simulink model "Lcontainer_simNN"  (R2018b)
settings: Solver=FixedStepAuto  StartTime=0.0  StopTime=600  FixedStep=0.1  RelTol=1e-3
libraries: neural x88, simulink x1
(part 3 of 4)

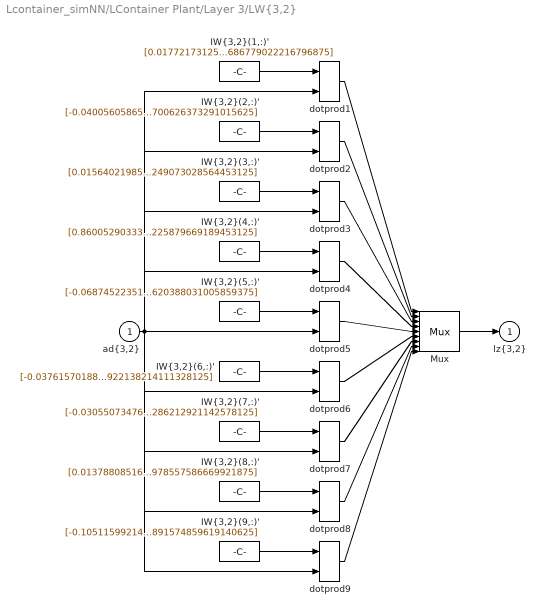
== system Lcontainer_simNN/LContainer Plant/Layer 3/LW{3,2} ==
  "ad{3,2}" : Inport  PortDimensions=10
      mask Display: e = 0.06;c1 = [120 230 180]/255;c2 = ([120 230 180]+0)/(256+128);c3 = ([120 230 180]+128)/(256+128);patch([0 1 1 0],[0 0 1 1],c1);patch([0 1 1 1-e 1-e 0+e],[0 0 1 1-e 0+e 0+e],c2);patch([0 0 1 1-e 0+e 0+e],[0 1 1 1-e 1-e 0+e],c3);plot([0 1 1 0 0],[0 0 1 1 0]);
  "IW{3,2}(1,:)'" : Constant  Value=[0.017721731250787138567392986487902817316353321075439453125;3.000123587276951301099561015566332824954398723004377058654057464082143269479274749755859375e-18;0.006631368793965075440766110403956190566532313823699951171875;0.0005830819266561507348278770024307959829457104206085205078125;-0.00058009248650328962791655751374264582409523427486419677734375;0.00089743107072331150531052657015607110224664211273193359375;0.000417621773328847646113148872615283835330046713352203369140625;-2.208352547409586067716440764973830234430475893202518079155068780883297563377709593623876571655273438e-21;0.00013978297890123654351364479442310084778000600636005401611328125;0.000674010021193850554499515936868192511610686779022216796875]
      mask Display: e = 0.06;c1 = [120 150 230]/255;c2 = ([120 150 230]+0)/383;c3 = ([120 150 230]+128)/383;patch([0 1 1 0],[0 0 1 1],c1);patch([0 1 1 1-e 1-e 0+e],[0 0 1 1-e 0+e 0+e],c2);patch([0 0 1 1-e 0+e 0+e],[0 1 1 1-e 1-e 0+e],c3);plot([0 1 1 0 0],[0 0 1 1 0]);disp('weights');
  "IW{3,2}(2,:)'" : Constant  Value=[-0.04005605865106844076795056253104121424257755279541015625;-3.29867064884893000845695736657715495575445867532972388236345295808860100805759429931640625e-17;0.06916512907204268312266748353067669086158275604248046875;-0.042226033791083257551424168241283041425049304962158203125;0.034903285783379846274332436451004468835890293121337890625;-0.0021373573678505207625033524010405017179436981678009033203125;-0.003622572133452827032595866540987117332406342029571533203125;2.9787149770187764768538925291780095327185039558298075188479125952056847381754778325557708740234375e-22;0.0435714010459078426862333799363113939762115478515625;0.000252495443577469718711425716861640466959215700626373291015625]
      mask Display: e = 0.06;c1 = [120 150 230]/255;c2 = ([120 150 230]+0)/383;c3 = ([120 150 230]+128)/383;patch([0 1 1 0],[0 0 1 1],c1);patch([0 1 1 1-e 1-e 0+e],[0 0 1 1-e 0+e 0+e],c2);patch([0 0 1 1-e 0+e 0+e],[0 1 1 1-e 1-e 0+e],c3);plot([0 1 1 0 0],[0 0 1 1 0]);disp('weights');
  "IW{3,2}(3,:)'" : Constant  Value=[0.0156402198576308069932760957954087643884122371673583984375;-2.7705357247132681851359167346903580323963177435846357010706952905820799060165882110595703125e-17;0.005717664581344373588012164333349574008025228977203369140625;0.001120727306336578681100757393096500891260802745819091796875;-0.0010906626797669602239870823012779510463587939739227294921875;0.000717501659741846928471098454593857240979559719562530517578125;0.00049104555462250770898890994686780686606653034687042236328125;-8.808503989752254956010719320420912897565545125168497871668595033955995177166187204420566558837890625e-22;0.00025255883377770980101340025925082954927347600460052490234375;-0.00104828749438158792817166187205657479353249073028564453125]
      mask Display: e = 0.06;c1 = [120 150 230]/255;c2 = ([120 150 230]+0)/383;c3 = ([120 150 230]+128)/383;patch([0 1 1 0],[0 0 1 1],c1);patch([0 1 1 1-e 1-e 0+e],[0 0 1 1-e 0+e 0+e],c2);patch([0 0 1 1-e 0+e 0+e],[0 1 1 1-e 1-e 0+e],c3);plot([0 1 1 0 0],[0 0 1 1 0]);disp('weights');
  "IW{3,2}(4,:)'" : Constant  Value=[0.86005290333067818675516491566668264567852020263671875;1.08054859226237535721582342014765368435526095617325859077340055591776035726070404052734375e-16;0.4392103630130466118686172194429673254489898681640625;0.0309526769540591877027946310363404336385428905487060546875;-0.030153085840038874876345431630397797562181949615478515625;0.025833991374961805254084623584276414476335048675537109375;-0.0286867731698114518390507754475038382224738597869873046875;1.04433448485527096216197080488959096762601167281087898865664376213402420034981332719326019287109375e-20;0.01039470392753527594464912908733822405338287353515625;-0.00160357287137106942383202312640833042678423225879669189453125]
      mask Display: e = 0.06;c1 = [120 150 230]/255;c2 = ([120 150 230]+0)/383;c3 = ([120 150 230]+128)/383;patch([0 1 1 0],[0 0 1 1],c1);patch([0 1 1 1-e 1-e 0+e],[0 0 1 1-e 0+e 0+e],c2);patch([0 0 1 1-e 0+e 0+e],[0 1 1 1-e 1-e 0+e],c3);plot([0 1 1 0 0],[0 0 1 1 0]);disp('weights');
  "IW{3,2}(5,:)'" : Constant  Value=[-0.0687452235173775239029936301449197344481945037841796875;-2.0902295329942603015523256376234939712702367786635766766512034564584610052406787872314453125e-17;-0.1778346260095364506081949684812570922076702117919921875;0.37951707531323919386778698026319034397602081298828125;-0.25677471515412253477705917248385958373546600341796875;0.282905692872918612668087234851554967463016510009765625;0.28903582809806682707431946255383081734180450439453125;1.168985956367130130783772982847233629991089391960804043152279824147043996163120027631521224975585938e-21;0.298430584822482192208781270892359316349029541015625;0.270396007685359263117419459376833401620388031005859375]
      mask Display: e = 0.06;c1 = [120 150 230]/255;c2 = ([120 150 230]+0)/383;c3 = ([120 150 230]+128)/383;patch([0 1 1 0],[0 0 1 1],c1);patch([0 1 1 1-e 1-e 0+e],[0 0 1 1-e 0+e 0+e],c2);patch([0 0 1 1-e 0+e 0+e],[0 1 1 1-e 1-e 0+e],c3);plot([0 1 1 0 0],[0 0 1 1 0]);disp('weights');
  "IW{3,2}(6,:)'" : Constant  Value=[-0.037615701889427345661065515969312400557100772857666015625;-2.0255214901096142112965294281557460666901378224425030183386553517266293056309223175048828125e-17;-0.018940509565756220855536895442128297872841358184814453125;-0.0011494809468569548542571379101673301192931830883026123046875;0.0003933836267355390338938680994118612943566404283046722412109375;-0.00270488027420923322907686525695680757053196430206298828125;-0.0035495085585161519937946739133849405334331095218658447265625;2.771026078124981596591574202811655532744747077067631470356952327893651499834959395229816436767578125e-21;-0.005884709230925987653859632331432294449768960475921630859375;-0.002282368848335381006364741551806218922138214111328125]
      mask Display: e = 0.06;c1 = [120 150 230]/255;c2 = ([120 150 230]+0)/383;c3 = ([120 150 230]+128)/383;patch([0 1 1 0],[0 0 1 1],c1);patch([0 1 1 1-e 1-e 0+e],[0 0 1 1-e 0+e 0+e],c2);patch([0 0 1 1-e 0+e 0+e],[0 1 1 1-e 1-e 0+e],c3);plot([0 1 1 0 0],[0 0 1 1 0]);disp('weights');
  "IW{3,2}(7,:)'" : Constant  Value=[-0.0305507347678967249027248698212133604101836681365966796875;2.7496360392653631819364899496901638274924214552417077450652271863873465918004512786865234375e-17;0.0037154083625400755562517840502323451801203191280364990234375;-0.0117954745462954015133849594576531671918928623199462890625;0.00873441603258174291413151735241626738570630550384521484375;-0.00256346476134278015990286547776122461073100566864013671875;-0.0002901674951942543917611516679500027748872525990009307861328125;2.874094316443142059162815388265592867958623516934298226354737443299924848361115437000989913940429688e-21;0.009189198861728177514240911705201142467558383941650390625;-0.0149119845092046850176803474141706828959286212921142578125]
      mask Display: e = 0.06;c1 = [120 150 230]/255;c2 = ([120 150 230]+0)/383;c3 = ([120 150 230]+128)/383;patch([0 1 1 0],[0 0 1 1],c1);patch([0 1 1 1-e 1-e 0+e],[0 0 1 1-e 0+e 0+e],c2);patch([0 0 1 1-e 0+e 0+e],[0 1 1 1-e 1-e 0+e],c3);plot([0 1 1 0 0],[0 0 1 1 0]);disp('weights');
  "IW{3,2}(8,:)'" : Constant  Value=[0.01378808516196154514144023295330043765716254711151123046875;-4.899238598294270608298336688091797164883411976597261949795125701712095178663730621337890625e-17;-0.02461851504914606969531831737185711972415447235107421875;0.053656095043096409258343015835635014809668064117431640625;-0.06243497389268269637252473103217198513448238372802734375;-0.006117530417972946547855439547447531367652118206024169921875;0.005742975335650324364422658618423156440258026123046875;-1.090939145799021708153406170841651324421968177498445589848749190386989482703938847407698631286621094e-21;-0.00137001382693252723131427384117841938859783113002777099609375;0.03560214339080740308940420391081715933978557586669921875]
      mask Display: e = 0.06;c1 = [120 150 230]/255;c2 = ([120 150 230]+0)/383;c3 = ([120 150 230]+128)/383;patch([0 1 1 0],[0 0 1 1],c1);patch([0 1 1 1-e 1-e 0+e],[0 0 1 1-e 0+e 0+e],c2);patch([0 0 1 1-e 0+e 0+e],[0 1 1 1-e 1-e 0+e],c3);plot([0 1 1 0 0],[0 0 1 1 0]);disp('weights');
  "IW{3,2}(9,:)'" : Constant  Value=[-0.10511599214514828759536868574286927469074726104736328125;5.121980772139466446942862502458263931975946490625546669850365333331865258514881134033203125e-17;0.2601261896053455036081913931411691009998321533203125;-0.136425741683425361117087959428317844867706298828125;0.1081606731296494150473819217950222082436084747314453125;-0.0089247157820076909728879144267921219579875469207763671875;0.0011455689908133749425889202910866515594534575939178466796875;8.549650359076011053606725543058816108935553021266017400495596662013397804003034252673387527465820313e-22;0.1629678156227741536721254078656784258782863616943359375;0.83692845002217597372151658419170416891574859619140625]
      mask Display: e = 0.06;c1 = [120 150 230]/255;c2 = ([120 150 230]+0)/383;c3 = ([120 150 230]+128)/383;patch([0 1 1 0],[0 0 1 1],c1);patch([0 1 1 1-e 1-e 0+e],[0 0 1 1-e 0+e 0+e],c2);patch([0 0 1 1-e 0+e 0+e],[0 1 1 1-e 1-e 0+e],c3);plot([0 1 1 0 0],[0 0 1 1 0]);disp('weights');
  Mux : Mux  Inputs=9
      mask Display: e = 0.06;c1 = [120 150 230]/255;c2 = ([120 150 230]+0)/383;c3 = ([120 150 230]+128)/383;patch([0 1 1 0],[0 0 1 1],c1);patch([0 1 1 1-e 1-e 0+e],[0 0 1 1-e 0+e 0+e],c2);patch([0 0 1 1-e 0+e 0+e],[0 1 1 1-e 1-e 0+e],c3);plot([0 1 1 0 0],[0 0 1 1 0]);disp('Mux');
  dotprod{1..9} (9 alike) : neural/Weight Functions/dotprod
  "lz{3,2}" : Outport
      mask Display: e = 0.06;c1 = [120 230 180]/255;c2 = ([120 230 180]+0)/(256+128);c3 = ([120 230 180]+128)/(256+128);patch([0 1 1 0],[0 0 1 1],c1);patch([0 1 1 1-e 1-e 0+e],[0 0 1 1-e 0+e 0+e],c2);patch([0 0 1 1-e 0+e 0+e],[0 1 1 1-e 1-e 0+e],c3);plot([0 1 1 0 0],[0 0 1 1 0]);
  wires:
  Mux/1 -> "lz{3,2}"/1
  dotprod9/1 -> Mux/9
  "IW{3,2}(9,:)'"/1 -> dotprod9/1
  dotprod8/1 -> Mux/8
  "IW{3,2}(8,:)'"/1 -> dotprod8/1
  dotprod7/1 -> Mux/7
  "IW{3,2}(7,:)'"/1 -> dotprod7/1
  dotprod6/1 -> Mux/6
  "IW{3,2}(6,:)'"/1 -> dotprod6/1
  dotprod5/1 -> Mux/5
  "IW{3,2}(5,:)'"/1 -> dotprod5/1
  dotprod4/1 -> Mux/4
  "IW{3,2}(4,:)'"/1 -> dotprod4/1
  dotprod3/1 -> Mux/3
  "IW{3,2}(3,:)'"/1 -> dotprod3/1
  dotprod2/1 -> Mux/2
  "IW{3,2}(2,:)'"/1 -> dotprod2/1
  dotprod1/1 -> Mux/1
  "ad{3,2}"/1 -> dotprod9/2, dotprod8/2, dotprod7/2, dotprod6/2, dotprod5/2, dotprod4/2, dotprod3/2, dotprod2/2, dotprod1/2
  "IW{3,2}(1,:)'"/1 -> dotprod1/1

== system Lcontainer_simNN/LContainer tr/Layer 1/Delays 1 ==
  "p{1}" : Inport  PortDimensions=19
      mask Display: e = 0.06;c1 = [120 230 180]/255;c2 = ([120 230 180]+0)/(256+128);c3 = ([120 230 180]+128)/(256+128);patch([0 1 1 0],[0 0 1 1],c1);patch([0 1 1 1-e 1-e 0+e],[0 0 1 1-e 0+e 0+e],c2);patch([0 0 1 1-e 0+e 0+e],[0 1 1 1-e 1-e 0+e],c3);plot([0 1 1 0 0],[0 0 1 1 0]);
  mux : Mux  Inputs=1
      mask Display: e = 0.06;c1 = [120 150 230]/255;c2 = ([120 150 230]+0)/383;c3 = ([120 150 230]+128)/383;patch([0 1 1 0],[0 0 1 1],c1);patch([0 1 1 1-e 1-e 0+e],[0 0 1 1-e 0+e 0+e],c2);patch([0 0 1 1-e 0+e 0+e],[0 1 1 1-e 1-e 0+e],c3);plot([0 1 1 0 0],[0 0 1 1 0]);disp('Mux')
  "pd{1,1}" : Outport
      mask Display: e = 0.06;c1 = [120 230 180]/255;c2 = ([120 230 180]+0)/(256+128);c3 = ([120 230 180]+128)/(256+128);patch([0 1 1 0],[0 0 1 1],c1);patch([0 1 1 1-e 1-e 0+e],[0 0 1 1-e 0+e 0+e],c2);patch([0 0 1 1-e 0+e 0+e],[0 1 1 1-e 1-e 0+e],c3);plot([0 1 1 0 0],[0 0 1 1 0]);
  wires:
  mux/1 -> "pd{1,1}"/1
  "p{1}"/1 -> mux/1

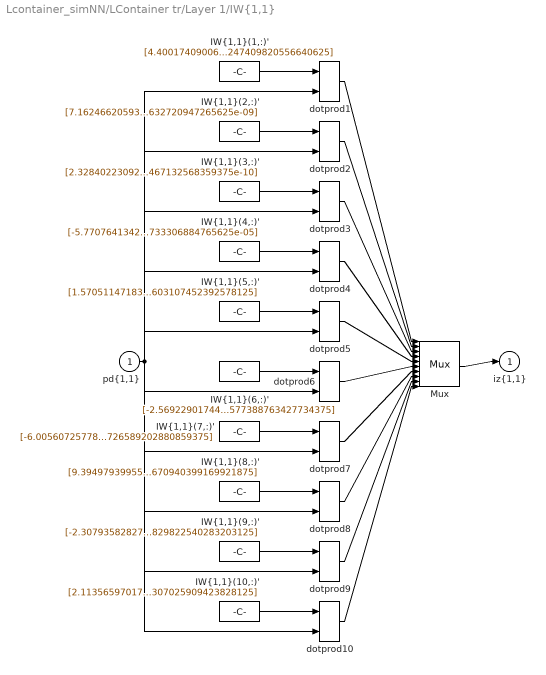
== system Lcontainer_simNN/LContainer tr/Layer 1/IW{1,1} ==
  "pd{1,1}" : Inport  PortDimensions=19
      mask Display: e = 0.06;c1 = [120 230 180]/255;c2 = ([120 230 180]+0)/(256+128);c3 = ([120 230 180]+128)/(256+128);patch([0 1 1 0],[0 0 1 1],c1);patch([0 1 1 1-e 1-e 0+e],[0 0 1 1-e 0+e 0+e],c2);patch([0 0 1 1-e 0+e 0+e],[0 1 1 1-e 1-e 0+e],c3);plot([0 1 1 0 0],[0 0 1 1 0]);
  "IW{1,1}(1,:)'" : Constant  Value=[4.40017409006617107452076869647701606869105717123602516949176788330078125e-09;0.01345267619395669640713908421503219869919121265411376953125;8.158769329916370116780044430271345845540054142475128173828125e-05;0.133282506165966319056082056704326532781124114990234375;0.118798799147599110082040851921192370355129241943359375;-0.00160146802195825096147563382231737705296836793422698974609375;0.00361362526321039496945974889285935205407440662384033203125;0.00402460725956179689311031921761241392232477664947509765625;0.1388328803151288315387290595026570372283458709716796875;0.13563305647747092574917360252584330737590789794921875;0.03992381222266881690696749274138710461556911468505859375;-0.0016005219135142756577139255824704378028400242328643798828125;0.433616038493515876250938845259952358901500701904296875;0.48731317755691783144555984108592383563518524169921875;0.0112602065374665973040979594088639714755117893218994140625;0.004024609800961928031404202243948020623065531253814697265625;-0.07276424533892690560410443367800326086580753326416015625;-0.036403357952666894059579050235697650350630283355712890625;0.0019376179722031734199705343968389570363797247409820556640625]
      mask Display: e = 0.06;c1 = [120 150 230]/255;c2 = ([120 150 230]+0)/383;c3 = ([120 150 230]+128)/383;patch([0 1 1 0],[0 0 1 1],c1);patch([0 1 1 1-e 1-e 0+e],[0 0 1 1-e 0+e 0+e],c2);patch([0 0 1 1-e 0+e 0+e],[0 1 1 1-e 1-e 0+e],c3);plot([0 1 1 0 0],[0 0 1 1 0]);disp('Weights');
  "IW{1,1}(10,:)'" : Constant  Value=[2.113565970177129623007061133470947840440334886125128832645714282989501953125e-10;0.03896513174368167187200384660172858275473117828369140625;-0.00069289406221726963612528304992110861348919570446014404296875;-0.00762248639883274237138977014183183200657367706298828125;0.383227265395797156433133068276220001280307769775390625;-0.0034013008372572842326342357210933187161572277545928955078125;0.003833531616325058961891603104277237434871494770050048828125;4.2035885052135081997419507882085554228979162871837615966796875e-05;0.26746096702046051607482013423577882349491119384765625;0.0134623389634068134357303136994232772849500179290771484375;0.061164726116837993263875006277885404415428638458251953125;-0.0034002204205467422004627309206625795923173427581787109375;-0.0004426065476116100398662478454525626148097217082977294921875;-0.0157469380460787157505198052831474342383444309234619140625;0.04609252485800897913836848829305381514132022857666015625;4.20365849119130210553678395068999407158116810023784637451171875e-05;-0.0927676528636662833804393812897615134716033935546875;-0.410080382762758655079693426159792579710483551025390625;0.00019232347600294465617305761373501127309282310307025909423828125]
      mask Display: e = 0.06;c1 = [120 150 230]/255;c2 = ([120 150 230]+0)/383;c3 = ([120 150 230]+128)/383;patch([0 1 1 0],[0 0 1 1],c1);patch([0 1 1 1-e 1-e 0+e],[0 0 1 1-e 0+e 0+e],c2);patch([0 0 1 1-e 0+e 0+e],[0 1 1 1-e 1-e 0+e],c3);plot([0 1 1 0 0],[0 0 1 1 0]);disp('Weights');
  "IW{1,1}(2,:)'" : Constant  Value=[7.1624662059342001339006781010011228050249343368705012835562229156494140625e-10;-8.999536615547740019975435916250137979854883951702504418790340423583984375e-10;-2.272043025698817149853437770521021044078935346988146193325519561767578125e-09;-5.42278631721199456096987225463094961508403457628446631133556365966796875e-09;5.8261390368475859080472936354401503056266165003762580454349517822265625e-09;5.78695274485159540658980997502973397939030064662802033126354217529296875e-09;-3.83991249249502824853957854315069687933803521673326031304895877838134765625e-10;3.119889020449836787037846329794475719321411588680348359048366546630859375e-09;3.79428320592626191941727236312149884600586347005446441471576690673828125e-09;4.0441135329039372901780793911376277183222782696248032152652740478515625e-09;3.0272237821613750687206104953048957373340499543701298534870147705078125e-09;2.992368260897594962679472776231719144401921539611066691577434539794921875e-09;-5.13434752897239199058995748141918935569805171326152049005031585693359375e-09;2.522088301447986899802429134362195817242735529362107627093791961669921875e-09;-3.80978185620454345008114858711807670932358860227395780384540557861328125e-09;5.4506060292929755970139896908456533797249221606762148439884185791015625e-09;-1.589321825348820627796800480382131970369385953745222650468349456787109375e-09;3.519654356750633884393332769598312925740657419737544842064380645751953125e-09;-4.28486277730642406559019761910257761972076195888803340494632720947265625e-09]
      mask Display: e = 0.06;c1 = [120 150 230]/255;c2 = ([120 150 230]+0)/383;c3 = ([120 150 230]+128)/383;patch([0 1 1 0],[0 0 1 1],c1);patch([0 1 1 1-e 1-e 0+e],[0 0 1 1-e 0+e 0+e],c2);patch([0 0 1 1-e 0+e 0+e],[0 1 1 1-e 1-e 0+e],c3);plot([0 1 1 0 0],[0 0 1 1 0]);disp('Weights');
  "IW{1,1}(3,:)'" : Constant  Value=[2.328402230929371488938198759394669623556950455167680047452449798583984375e-09;-3.09188994019135696677337519513127650494510589851415716111660003662109375e-09;-3.9808881126635397177467197427080947136346367187798023223876953125e-09;-3.319339377724885597549837556682374162253523763865814544260501861572265625e-09;4.91515374183487937575602001109668914846650977779063396155834197998046875e-09;3.27391084909379363396645737653740948491787321472656913101673126220703125e-09;-5.2136676587851719127595114843041861074635079376093926839530467987060546875e-10;-4.42383218663131527848705556484054657317983583197928965091705322265625e-10;-5.9657635190590810698770465468794566010757307594758458435535430908203125e-09;1.8256576634299592099538396390242568634310060815550968982279300689697265625e-09;-2.57527690285999316766621676359251547072659604964428581297397613525390625e-09;-3.410123602891442625652766509349554657770653420811868272721767425537109375e-09;-3.28398223063423191877047263554333100810112000544904731214046478271484375e-09;-2.6889830621702284196971282950977370773681940363530884496867656707763671875e-10;1.7612926143374152918424114727734101915057607357084634713828563690185546875e-09;-9.1113371902980798958826792068965531867785756503508309833705425262451171875e-10;3.75738764892813332766460044235862399120140509012344409711658954620361328125e-10;-4.81544049152883447916908949922899785267560446300194598734378814697265625e-09;6.2531053676675665477864397650241412573990373857668600976467132568359375e-10]
      mask Display: e = 0.06;c1 = [120 150 230]/255;c2 = ([120 150 230]+0)/383;c3 = ([120 150 230]+128)/383;patch([0 1 1 0],[0 0 1 1],c1);patch([0 1 1 1-e 1-e 0+e],[0 0 1 1-e 0+e 0+e],c2);patch([0 0 1 1-e 0+e 0+e],[0 1 1 1-e 1-e 0+e],c3);plot([0 1 1 0 0],[0 0 1 1 0]);disp('Weights');
  "IW{1,1}(4,:)'" : Constant  Value=[-5.7707641342750503806772659906522589257082955782607314176857471466064453125e-10;-0.00296619269589747970583548664080808521248400211334228515625;-3.65481476073493904583862172674724178023097920231521129608154296875e-06;0.002762072656014823157644144657751894555985927581787109375;-0.0090545077419806434260163285898670437745749950408935546875;0.000215452290449664953138342315952513672527857124805450439453125;-0.000696110597669588192400180748364846294862218201160430908203125;-0.0024990608335996420015512331502804954652674496173858642578125;-0.0167883714145944384910080771078355610370635986328125;0.004581902896608113819054697302135537029244005680084228515625;-0.004534723043989352143923188265262069762684404850006103515625;0.00021513843983774256119097245676385909973760135471820831298828125;0.0240123558391207962692259769710290129296481609344482421875;0.00568271731307086469531242300945450551807880401611328125;-0.000634410909431219207331442699882018132484517991542816162109375;-0.002499052787441458263473226253381653805263340473175048828125;0.0162818589674699164271398643677457584999501705169677734375;0.0163062017397326806944501953466897248290479183197021484375;6.5452257817100279271328722163758584429160691797733306884765625e-05]
      mask Display: e = 0.06;c1 = [120 150 230]/255;c2 = ([120 150 230]+0)/383;c3 = ([120 150 230]+128)/383;patch([0 1 1 0],[0 0 1 1],c1);patch([0 1 1 1-e 1-e 0+e],[0 0 1 1-e 0+e 0+e],c2);patch([0 0 1 1-e 0+e 0+e],[0 1 1 1-e 1-e 0+e],c3);plot([0 1 1 0 0],[0 0 1 1 0]);disp('Weights');
  "IW{1,1}(5,:)'" : Constant  Value=[1.57051147183871157788316781124537957481379635282792150974273681640625e-09;-0.0203196251152120456462402131592170917429029941558837890625;0.000281792887915606276270918950643817879608832299709320068359375;0.0286744668292554204247490901025230414234101772308349609375;-0.0274052653886996365473205372609299956820905208587646484375;0.00043645876558191516562945633239678500103764235973358154296875;-0.003829592790545395357415525694477764773182570934295654296875;-0.014778232753136687216422018309458508156239986419677734375;-0.0113428281769742712870030487692929455079138278961181640625;0.0308382918513680111260999439082297612912952899932861328125;-0.0268467963588808165853460963035104214213788509368896484375;0.0004350142461743746196030369066676257716608233749866485595703125;0.753704496154507186389537309878505766391754150390625;0.4102832936758271653587826222064904868602752685546875;-7.325478878100725337908782908158400459797121584415435791015625e-05;-0.0147782358891054323157820959977470920421183109283447265625;0.1025809329564021099567838746224879287183284759521484375;0.1857021251011930218499657030406524427235126495361328125;0.0004405501744805431882552604339053914372925646603107452392578125]
      mask Display: e = 0.06;c1 = [120 150 230]/255;c2 = ([120 150 230]+0)/383;c3 = ([120 150 230]+128)/383;patch([0 1 1 0],[0 0 1 1],c1);patch([0 1 1 1-e 1-e 0+e],[0 0 1 1-e 0+e 0+e],c2);patch([0 0 1 1-e 0+e 0+e],[0 1 1 1-e 1-e 0+e],c3);plot([0 1 1 0 0],[0 0 1 1 0]);disp('Weights');
  "IW{1,1}(6,:)'" : Constant  Value=[-2.5692290174429262391143412107806509592222710125497542321681976318359375e-09;-0.00776702788136899614779284917176482849754393100738525390625;0.0002875410507820698913401813445744892305810935795307159423828125;0.0125414266308371373515040403390230494551360607147216796875;-0.0814458250977431463812905576560297049582004547119140625;0.0002731458767526252274550346843540182817378081381320953369140625;-0.00132852876322621903104614915491765714250504970550537109375;0.01286707339226317477198779926084171165712177753448486328125;0.03500093650108358767081284668165608309209346771240234375;-0.01027299660668115448280968138305979664437472820281982421875;-0.0254587316253201585702914400144436513073742389678955078125;0.000274146747010343516497143934174118840019218623638153076171875;0.520031319096056154904772483860142529010772705078125;-0.73109112720811764152273326544673182070255279541015625;-0.00811748100756374234288070823595262481831014156341552734375;0.01286707743977752622932531068045136635191738605499267578125;0.026368614400726624047432977704374934546649456024169921875;0.06785457592044354113713922060924232937395572662353515625;-0.00014675430325078786856184132059155444949283264577388763427734375]
      mask Display: e = 0.06;c1 = [120 150 230]/255;c2 = ([120 150 230]+0)/383;c3 = ([120 150 230]+128)/383;patch([0 1 1 0],[0 0 1 1],c1);patch([0 1 1 1-e 1-e 0+e],[0 0 1 1-e 0+e 0+e],c2);patch([0 0 1 1-e 0+e 0+e],[0 1 1 1-e 1-e 0+e],c3);plot([0 1 1 0 0],[0 0 1 1 0]);disp('Weights');
  "IW{1,1}(7,:)'" : Constant  Value=[-6.00560725778598956991717326453668335251023790988256223499774932861328125e-09;0.043806778240186472483941315658739767968654632568359375;-0.000100138492794243937934750565688091228366829454898834228515625;0.0028577006213790149928566375336913552018813788890838623046875;0.1573122361947522918068642638900200836360454559326171875;-0.0028151321709028128727203554859670475707389414310455322265625;0.01011664157125011058446784062425649608485400676727294921875;0.03167278041242506392283218019656487740576267242431640625;0.286377220486189132397925050099729560315608978271484375;-0.00943356320441320235492543844202373293228447437286376953125;0.078451910448477268911204873802489601075649261474609375;-0.0028111375129141152710843254425299164722673594951629638671875;0.303387461615569564710170880061923526227474212646484375;-0.1334750480496697255805571558084920980036258697509765625;0.011175488822446448533565188654392841272056102752685546875;0.03167277451769272278436773149223881773650646209716796875;-0.2381577491621619524497788233929895795881748199462890625;-0.26266869111349733234561654171557165682315826416015625;-0.00013476915698231164086016986569660502937040291726589202880859375]
      mask Display: e = 0.06;c1 = [120 150 230]/255;c2 = ([120 150 230]+0)/383;c3 = ([120 150 230]+128)/383;patch([0 1 1 0],[0 0 1 1],c1);patch([0 1 1 1-e 1-e 0+e],[0 0 1 1-e 0+e 0+e],c2);patch([0 0 1 1-e 0+e 0+e],[0 1 1 1-e 1-e 0+e],c3);plot([0 1 1 0 0],[0 0 1 1 0]);disp('Weights');
  "IW{1,1}(8,:)'" : Constant  Value=[9.3949793995568735266368183057551777270788306850590743124485015869140625e-10;0.003065555585273392440182060880715653183870017528533935546875;-6.9910728012105853752811146506473960471339523792266845703125e-05;0.1102183158480669888934500022514839656651020050048828125;0.014925845011555520513990558129080454818904399871826171875;-0.00020009055553428986540774603408721077357768081128597259521484375;0.00018576964658563696369993067936121633465518243610858917236328125;0.0002477293251398351124625829555725431418977677822113037109375;0.0309111023775324837703504243791030603460967540740966796875;0.1100058492542145549553112005014554597437381744384765625;0.0011518027305354775445545012502179815783165395259857177734375;-0.000199965418539174537293501288104380364529788494110107421875;-0.00971029742272888109211326224112781346775591373443603515625;0.1439916375118344415984239503814023919403553009033203125;0.0019665903028653840788064766087472889921627938747406005859375;0.0002477247344637019898193341926884158965549431741237640380859375;-0.00590936207293043906652041385996199096553027629852294921875;-0.038156253507875680097694015557863167487084865570068359375;0.00157151653174637004166391829329540996695868670940399169921875]
      mask Display: e = 0.06;c1 = [120 150 230]/255;c2 = ([120 150 230]+0)/383;c3 = ([120 150 230]+128)/383;patch([0 1 1 0],[0 0 1 1],c1);patch([0 1 1 1-e 1-e 0+e],[0 0 1 1-e 0+e 0+e],c2);patch([0 0 1 1-e 0+e 0+e],[0 1 1 1-e 1-e 0+e],c3);plot([0 1 1 0 0],[0 0 1 1 0]);disp('Weights');
  "IW{1,1}(9,:)'" : Constant  Value=[-2.30793582827203089670661332048935687755175649726879782974720001220703125e-09;0.00847810682657990609401021941948783933185040950775146484375;-0.000823599797067461566503487890855694786296226084232330322265625;0.44088000479909894568919526136596687138080596923828125;0.055565439840595746978646474190099979750812053680419921875;0.0014469162529821967370924351570238286512903869152069091796875;0.000881155217338923011337337154458282384439371526241302490234375;-0.031353007196950631596532588218906312249600887298583984375;-0.11237303158152560367266659113738569431006908416748046875;0.49674157975532196029888609700719825923442840576171875;0.0173454646733493707266848815606863354332745075225830078125;0.001444677416220404610192051819694825098849833011627197265625;0.249057101693842153355973323414218612015247344970703125;-0.255818512424603461408167959234560839831829071044921875;0.005762235031577476844499852148828722420148551464080810546875;-0.031353005117842301652242298359851702116429805755615234375;-0.0259863898949828364681735592967015691101551055908203125;-0.1423119301351623289253467419257503934204578399658203125;0.007096302426458843577716795181231645983643829822540283203125]
      mask Display: e = 0.06;c1 = [120 150 230]/255;c2 = ([120 150 230]+0)/383;c3 = ([120 150 230]+128)/383;patch([0 1 1 0],[0 0 1 1],c1);patch([0 1 1 1-e 1-e 0+e],[0 0 1 1-e 0+e 0+e],c2);patch([0 0 1 1-e 0+e 0+e],[0 1 1 1-e 1-e 0+e],c3);plot([0 1 1 0 0],[0 0 1 1 0]);disp('Weights');
  Mux : Mux  Inputs=10
      mask Display: e = 0.06;c1 = [120 150 230]/255;c2 = ([120 150 230]+0)/383;c3 = ([120 150 230]+128)/383;patch([0 1 1 0],[0 0 1 1],c1);patch([0 1 1 1-e 1-e 0+e],[0 0 1 1-e 0+e 0+e],c2);patch([0 0 1 1-e 0+e 0+e],[0 1 1 1-e 1-e 0+e],c3);plot([0 1 1 0 0],[0 0 1 1 0]);disp('Mux');
  dotprod{1..10} (10 alike) : neural/Weight Functions/dotprod
  "iz{1,1}" : Outport
      mask Display: e = 0.06;c1 = [120 230 180]/255;c2 = ([120 230 180]+0)/(256+128);c3 = ([120 230 180]+128)/(256+128);patch([0 1 1 0],[0 0 1 1],c1);patch([0 1 1 1-e 1-e 0+e],[0 0 1 1-e 0+e 0+e],c2);patch([0 0 1 1-e 0+e 0+e],[0 1 1 1-e 1-e 0+e],c3);plot([0 1 1 0 0],[0 0 1 1 0]);
  wires:
  Mux/1 -> "iz{1,1}"/1
  dotprod10/1 -> Mux/10
  "IW{1,1}(10,:)'"/1 -> dotprod10/1
  dotprod9/1 -> Mux/9
  "IW{1,1}(9,:)'"/1 -> dotprod9/1
  dotprod8/1 -> Mux/8
  "IW{1,1}(8,:)'"/1 -> dotprod8/1
  dotprod7/1 -> Mux/7
  "IW{1,1}(7,:)'"/1 -> dotprod7/1
  dotprod6/1 -> Mux/6
  "IW{1,1}(6,:)'"/1 -> dotprod6/1
  dotprod5/1 -> Mux/5
  "IW{1,1}(5,:)'"/1 -> dotprod5/1
  dotprod4/1 -> Mux/4
  "IW{1,1}(4,:)'"/1 -> dotprod4/1
  dotprod3/1 -> Mux/3
  "IW{1,1}(3,:)'"/1 -> dotprod3/1
  dotprod2/1 -> Mux/2
  "IW{1,1}(2,:)'"/1 -> dotprod2/1
  dotprod1/1 -> Mux/1
  "pd{1,1}"/1 -> dotprod10/2, dotprod9/2, dotprod8/2, dotprod7/2, dotprod6/2, dotprod5/2, dotprod4/2, dotprod3/2, dotprod2/2, dotprod1/2
  "IW{1,1}(1,:)'"/1 -> dotprod1/1

== system Lcontainer_simNN/LContainer tr/Layer 2/Delays 1 ==
  "p{2}" : Inport  PortDimensions=10
      mask Display: e = 0.06;c1 = [120 230 180]/255;c2 = ([120 230 180]+0)/(256+128);c3 = ([120 230 180]+128)/(256+128);patch([0 1 1 0],[0 0 1 1],c1);patch([0 1 1 1-e 1-e 0+e],[0 0 1 1-e 0+e 0+e],c2);patch([0 0 1 1-e 0+e 0+e],[0 1 1 1-e 1-e 0+e],c3);plot([0 1 1 0 0],[0 0 1 1 0]);
  mux : Mux  Inputs=1
      mask Display: e = 0.06;c1 = [120 150 230]/255;c2 = ([120 150 230]+0)/383;c3 = ([120 150 230]+128)/383;patch([0 1 1 0],[0 0 1 1],c1);patch([0 1 1 1-e 1-e 0+e],[0 0 1 1-e 0+e 0+e],c2);patch([0 0 1 1-e 0+e 0+e],[0 1 1 1-e 1-e 0+e],c3);plot([0 1 1 0 0],[0 0 1 1 0]);disp('Mux')
  "pd{2,1}" : Outport
      mask Display: e = 0.06;c1 = [120 230 180]/255;c2 = ([120 230 180]+0)/(256+128);c3 = ([120 230 180]+128)/(256+128);patch([0 1 1 0],[0 0 1 1],c1);patch([0 1 1 1-e 1-e 0+e],[0 0 1 1-e 0+e 0+e],c2);patch([0 0 1 1-e 0+e 0+e],[0 1 1 1-e 1-e 0+e],c3);plot([0 1 1 0 0],[0 0 1 1 0]);
  wires:
  mux/1 -> "pd{2,1}"/1
  "p{2}"/1 -> mux/1

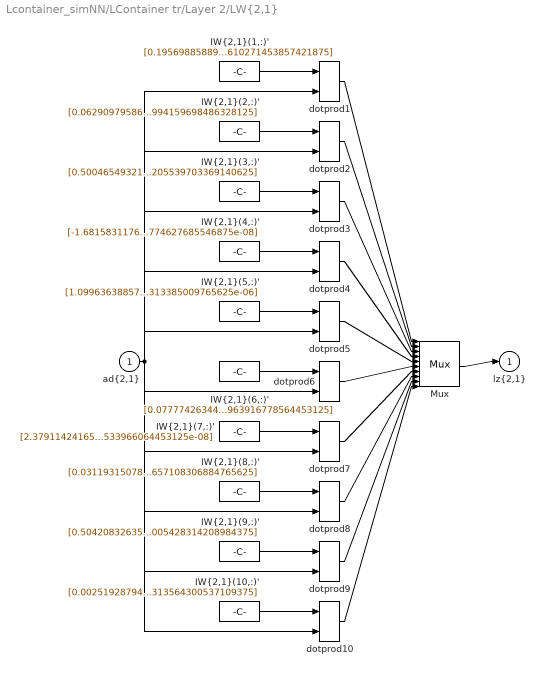
== system Lcontainer_simNN/LContainer tr/Layer 2/LW{2,1} ==
  "ad{2,1}" : Inport  PortDimensions=10
      mask Display: e = 0.06;c1 = [120 230 180]/255;c2 = ([120 230 180]+0)/(256+128);c3 = ([120 230 180]+128)/(256+128);patch([0 1 1 0],[0 0 1 1],c1);patch([0 1 1 1-e 1-e 0+e],[0 0 1 1-e 0+e 0+e],c2);patch([0 0 1 1-e 0+e 0+e],[0 1 1 1-e 1-e 0+e],c3);plot([0 1 1 0 0],[0 0 1 1 0]);
  "IW{2,1}(1,:)'" : Constant  Value=[0.195698858894761962279318368018721230328083038330078125;3.364753922179192513152566030112423922648900997955934144556522369384765625e-09;-2.568646250412722035674146820079244424306352811981923878192901611328125e-09;0.0218466171238021304723542215242559905163943767547607421875;0.1649320777576779584183697124899481423199176788330078125;-0.400923473566163923731409113315748982131481170654296875;-0.0275292125962848695241991237026013550348579883575439453125;0.04957881151029570887533992618045886047184467315673828125;0.79181222093064906886183962342329323291778564453125;0.1444341266512274568611928771133534610271453857421875]
      mask Display: e = 0.06;c1 = [120 150 230]/255;c2 = ([120 150 230]+0)/383;c3 = ([120 150 230]+128)/383;patch([0 1 1 0],[0 0 1 1],c1);patch([0 1 1 1-e 1-e 0+e],[0 0 1 1-e 0+e 0+e],c2);patch([0 0 1 1-e 0+e 0+e],[0 1 1 1-e 1-e 0+e],c3);plot([0 1 1 0 0],[0 0 1 1 0]);disp('weights');
  "IW{2,1}(10,:)'" : Constant  Value=[0.00251928794107436453131310116759777883999049663543701171875;-4.426563548358155215715667549387923873638328586821444332599639892578125e-09;-3.409078853940243439779187858084362472421702250358066521584987640380859375e-09;-0.00037792446119817748977076643512873488361947238445281982421875;-0.0027757359356523707803743317157341152778826653957366943359375;0.0001342860664289106660367056900184934420394711196422576904296875;0.00889341695673535881372373523845453746616840362548828125;0.00118984046504649909094253334984614411951042711734771728515625;0.006928439120522493673004493786038437974639236927032470703125;0.001754388305545986036226846493946140981279313564300537109375]
      mask Display: e = 0.06;c1 = [120 150 230]/255;c2 = ([120 150 230]+0)/383;c3 = ([120 150 230]+128)/383;patch([0 1 1 0],[0 0 1 1],c1);patch([0 1 1 1-e 1-e 0+e],[0 0 1 1-e 0+e 0+e],c2);patch([0 0 1 1-e 0+e 0+e],[0 1 1 1-e 1-e 0+e],c3);plot([0 1 1 0 0],[0 0 1 1 0]);disp('weights');
  "IW{2,1}(2,:)'" : Constant  Value=[0.062909795862125805765430186511366628110408782958984375;4.85216656451100071088621719915014163237998445765697397291660308837890625e-09;1.393789994876343612722053750554128404015585829256451688706874847412109375e-09;0.0132537332777675730122179942327420576475560665130615234375;0.1507742074580266378180937181241461075842380523681640625;-0.098047743326234615413028450348065234720706939697265625;-0.06957658701374734577793645939891575835645198822021484375;-0.12321059722953621451413397380747483111917972564697265625;0.2292392155051094226880792348310933448374271392822265625;0.210312052982961461555788673649658448994159698486328125]
      mask Display: e = 0.06;c1 = [120 150 230]/255;c2 = ([120 150 230]+0)/383;c3 = ([120 150 230]+128)/383;patch([0 1 1 0],[0 0 1 1],c1);patch([0 1 1 1-e 1-e 0+e],[0 0 1 1-e 0+e 0+e],c2);patch([0 0 1 1-e 0+e 0+e],[0 1 1 1-e 1-e 0+e],c3);plot([0 1 1 0 0],[0 0 1 1 0]);disp('weights');
  "IW{2,1}(3,:)'" : Constant  Value=[0.500465493214111489805873134173452854156494140625;-3.19079372666514791766735888536334064813360100743011571466922760009765625e-09;-2.152556527473783284307865803770647150638950506618130020797252655029296875e-09;-0.021421631987128368634909492129736463539302349090576171875;0.260454007048182167860517211011028848588466644287109375;-0.1342362164434130200607597771522705443203449249267578125;0.48567024136403069700662626928533427417278289794921875;0.06707178334271797492949218622015905566513538360595703125;-0.173800926672021016639035906337085179984569549560546875;0.41955871811106748570097124684252776205539703369140625]
      mask Display: e = 0.06;c1 = [120 150 230]/255;c2 = ([120 150 230]+0)/383;c3 = ([120 150 230]+128)/383;patch([0 1 1 0],[0 0 1 1],c1);patch([0 1 1 1-e 1-e 0+e],[0 0 1 1-e 0+e 0+e],c2);patch([0 0 1 1-e 0+e 0+e],[0 1 1 1-e 1-e 0+e],c3);plot([0 1 1 0 0],[0 0 1 1 0]);disp('weights');
  "IW{2,1}(4,:)'" : Constant  Value=[-1.681583117658367056675294153901545346485590926022268831729888916015625e-08;-4.64183582891435646917291184786191760025531038991175591945648193359375e-09;-5.2191431800173359806393363381771255404828480095602571964263916015625e-10;-1.28600029720050548333913634159626770969708786651608534157276153564453125e-08;-1.2550299604320515973595261648154686184852835140191018581390380859375e-08;2.456900535475159499050901507001716528311163756370660848915576934814453125e-09;-6.0106192673240309381229210081327984926957697098259814083576202392578125e-09;-1.54632567835267709216418539897031081409295438788831233978271484375e-08;-2.9385676863732398853714766588651752243777082185260951519012451171875e-08;-3.71109889763679068822377414386959326719761520507745444774627685546875e-08]
      mask Display: e = 0.06;c1 = [120 150 230]/255;c2 = ([120 150 230]+0)/383;c3 = ([120 150 230]+128)/383;patch([0 1 1 0],[0 0 1 1],c1);patch([0 1 1 1-e 1-e 0+e],[0 0 1 1-e 0+e 0+e],c2);patch([0 0 1 1-e 0+e 0+e],[0 1 1 1-e 1-e 0+e],c3);plot([0 1 1 0 0],[0 0 1 1 0]);disp('weights');
  "IW{2,1}(5,:)'" : Constant  Value=[1.099636388572747640866335283593713256777846254408359527587890625e-05;-3.423743288183268992105220377038243828593522266601212322711944580078125e-09;-6.8401046571147334968893574281699650196930662104932707734405994415283203125e-10;5.367878215521328825611644015858292533494022791273891925811767578125e-07;1.982594018795957437691253322231688116517034359276294708251953125e-05;1.26111212175133405484495074944106818293221294879913330078125e-05;8.42883854642876420896167866114723210557713173329830169677734375e-06;-2.05108325997118434995576674584327747652423568069934844970703125e-06;7.46628678827483881639474720681715069758865865878760814666748046875e-07;7.94594249356735484769720390119118746952153742313385009765625e-06]
      mask Display: e = 0.06;c1 = [120 150 230]/255;c2 = ([120 150 230]+0)/383;c3 = ([120 150 230]+128)/383;patch([0 1 1 0],[0 0 1 1],c1);patch([0 1 1 1-e 1-e 0+e],[0 0 1 1-e 0+e 0+e],c2);patch([0 0 1 1-e 0+e 0+e],[0 1 1 1-e 1-e 0+e],c3);plot([0 1 1 0 0],[0 0 1 1 0]);disp('weights');
  "IW{2,1}(6,:)'" : Constant  Value=[0.0777742634472124994005071130231954157352447509765625;-2.422349663184710033616213359125741988453484054844011552631855010986328125e-09;4.01639945478776454009496262899381324729120024130679666996002197265625e-09;0.03153712074940352716456715143067413009703159332275390625;0.53582477329683175781838144757784903049468994140625;0.77409014455006441846052211985806934535503387451171875;0.10588721130393539959779758419244899414479732513427734375;0.048860266895737407277788832971054944209754467010498046875;0.1185473857292629329407418481423519551753997802734375;-0.172824370655559722553817891821381635963916778564453125]
      mask Display: e = 0.06;c1 = [120 150 230]/255;c2 = ([120 150 230]+0)/383;c3 = ([120 150 230]+128)/383;patch([0 1 1 0],[0 0 1 1],c1);patch([0 1 1 1-e 1-e 0+e],[0 0 1 1-e 0+e 0+e],c2);patch([0 0 1 1-e 0+e 0+e],[0 1 1 1-e 1-e 0+e],c3);plot([0 1 1 0 0],[0 0 1 1 0]);disp('weights');
  "IW{2,1}(7,:)'" : Constant  Value=[2.379114241653396747514466794647114422645017839386127889156341552734375e-08;4.6882953715594181424291758491194881397490235031000338494777679443359375e-09;-9.0150367369742511557755539755641509269690203609570744447410106658935546875e-10;-2.65704727287802447663307304896208871358709302512579597532749176025390625e-09;-1.1483337616841846668913032676606622572990090702660381793975830078125e-08;4.26139652523061414622805860943390021677856793758110143244266510009765625e-09;3.1212686929624802720904135945600987867010189802385866641998291015625e-08;4.038651237970575862670089060772748990046920880558900535106658935546875e-08;2.3342902694173964847576213210537943165689966917852871119976043701171875e-08;-9.0283573687523543257961618213602861260369536466896533966064453125e-08]
      mask Display: e = 0.06;c1 = [120 150 230]/255;c2 = ([120 150 230]+0)/383;c3 = ([120 150 230]+128)/383;patch([0 1 1 0],[0 0 1 1],c1);patch([0 1 1 1-e 1-e 0+e],[0 0 1 1-e 0+e 0+e],c2);patch([0 0 1 1-e 0+e 0+e],[0 1 1 1-e 1-e 0+e],c3);plot([0 1 1 0 0],[0 0 1 1 0]);disp('weights');
  "IW{2,1}(8,:)'" : Constant  Value=[0.0311931507843391832290880216760342591442167758941650390625;5.283600843470311617276317735680986331647801534927566535770893096923828125e-10;-1.88865707469585051593369005363577672884645153317251242697238922119140625e-09;-0.01171534691780429758567461107077178894542157649993896484375;-0.02111806227127561996770310770443757064640522003173828125;0.333991863330524996200665555079467594623565673828125;0.360541833768206476662498971563763916492462158203125;-0.0789544868590297543864409135494497604668140411376953125;0.04745974599241149782802295931105618365108966827392578125;0.44488627535968439108415850569144822657108306884765625]
      mask Display: e = 0.06;c1 = [120 150 230]/255;c2 = ([120 150 230]+0)/383;c3 = ([120 150 230]+128)/383;patch([0 1 1 0],[0 0 1 1],c1);patch([0 1 1 1-e 1-e 0+e],[0 0 1 1-e 0+e 0+e],c2);patch([0 0 1 1-e 0+e 0+e],[0 1 1 1-e 1-e 0+e],c3);plot([0 1 1 0 0],[0 0 1 1 0]);disp('weights');
  "IW{2,1}(9,:)'" : Constant  Value=[0.5042083263591956576732400208129547536373138427734375;-2.610664124473003883905085237304190270979376009563566185534000396728515625e-09;2.141664514886540781802744056621680412977326568579883314669132232666015625e-09;0.0160616519821773044707224897820196929387748241424560546875;0.6671477657835473973335638220305554568767547607421875;-0.2044712599111734030454812227617367170751094818115234375;-0.1332900168677327024102652330839191563427448272705078125;-0.0322048568688966252437921866658143699169158935546875;-0.1543782216720164524037528508415562100708484649658203125;-0.212638985297296245757792121366946958005428314208984375]
      mask Display: e = 0.06;c1 = [120 150 230]/255;c2 = ([120 150 230]+0)/383;c3 = ([120 150 230]+128)/383;patch([0 1 1 0],[0 0 1 1],c1);patch([0 1 1 1-e 1-e 0+e],[0 0 1 1-e 0+e 0+e],c2);patch([0 0 1 1-e 0+e 0+e],[0 1 1 1-e 1-e 0+e],c3);plot([0 1 1 0 0],[0 0 1 1 0]);disp('weights');
  Mux : Mux  Inputs=10
      mask Display: e = 0.06;c1 = [120 150 230]/255;c2 = ([120 150 230]+0)/383;c3 = ([120 150 230]+128)/383;patch([0 1 1 0],[0 0 1 1],c1);patch([0 1 1 1-e 1-e 0+e],[0 0 1 1-e 0+e 0+e],c2);patch([0 0 1 1-e 0+e 0+e],[0 1 1 1-e 1-e 0+e],c3);plot([0 1 1 0 0],[0 0 1 1 0]);disp('Mux');
  dotprod{1..10} (10 alike) : neural/Weight Functions/dotprod
  "lz{2,1}" : Outport
      mask Display: e = 0.06;c1 = [120 230 180]/255;c2 = ([120 230 180]+0)/(256+128);c3 = ([120 230 180]+128)/(256+128);patch([0 1 1 0],[0 0 1 1],c1);patch([0 1 1 1-e 1-e 0+e],[0 0 1 1-e 0+e 0+e],c2);patch([0 0 1 1-e 0+e 0+e],[0 1 1 1-e 1-e 0+e],c3);plot([0 1 1 0 0],[0 0 1 1 0]);
  wires:
  Mux/1 -> "lz{2,1}"/1
  dotprod10/1 -> Mux/10
  "IW{2,1}(10,:)'"/1 -> dotprod10/1
  dotprod9/1 -> Mux/9
  "IW{2,1}(9,:)'"/1 -> dotprod9/1
  dotprod8/1 -> Mux/8
  "IW{2,1}(8,:)'"/1 -> dotprod8/1
  dotprod7/1 -> Mux/7
  "IW{2,1}(7,:)'"/1 -> dotprod7/1
  dotprod6/1 -> Mux/6
  "IW{2,1}(6,:)'"/1 -> dotprod6/1
  dotprod5/1 -> Mux/5
  "IW{2,1}(5,:)'"/1 -> dotprod5/1
  dotprod4/1 -> Mux/4
  "IW{2,1}(4,:)'"/1 -> dotprod4/1
  dotprod3/1 -> Mux/3
  "IW{2,1}(3,:)'"/1 -> dotprod3/1
  dotprod2/1 -> Mux/2
  "IW{2,1}(2,:)'"/1 -> dotprod2/1
  dotprod1/1 -> Mux/1
  "ad{2,1}"/1 -> dotprod10/2, dotprod9/2, dotprod8/2, dotprod7/2, dotprod6/2, dotprod5/2, dotprod4/2, dotprod3/2, dotprod2/2, dotprod1/2
  "IW{2,1}(1,:)'"/1 -> dotprod1/1

== system Lcontainer_simNN/LContainer tr/Layer 3/Delays 1 ==
  "p{3}" : Inport  PortDimensions=10
      mask Display: e = 0.06;c1 = [120 230 180]/255;c2 = ([120 230 180]+0)/(256+128);c3 = ([120 230 180]+128)/(256+128);patch([0 1 1 0],[0 0 1 1],c1);patch([0 1 1 1-e 1-e 0+e],[0 0 1 1-e 0+e 0+e],c2);patch([0 0 1 1-e 0+e 0+e],[0 1 1 1-e 1-e 0+e],c3);plot([0 1 1 0 0],[0 0 1 1 0]);
  mux : Mux  Inputs=1
      mask Display: e = 0.06;c1 = [120 150 230]/255;c2 = ([120 150 230]+0)/383;c3 = ([120 150 230]+128)/383;patch([0 1 1 0],[0 0 1 1],c1);patch([0 1 1 1-e 1-e 0+e],[0 0 1 1-e 0+e 0+e],c2);patch([0 0 1 1-e 0+e 0+e],[0 1 1 1-e 1-e 0+e],c3);plot([0 1 1 0 0],[0 0 1 1 0]);disp('Mux')
  "pd{3,2}" : Outport
      mask Display: e = 0.06;c1 = [120 230 180]/255;c2 = ([120 230 180]+0)/(256+128);c3 = ([120 230 180]+128)/(256+128);patch([0 1 1 0],[0 0 1 1],c1);patch([0 1 1 1-e 1-e 0+e],[0 0 1 1-e 0+e 0+e],c2);patch([0 0 1 1-e 0+e 0+e],[0 1 1 1-e 1-e 0+e],c3);plot([0 1 1 0 0],[0 0 1 1 0]);
  wires:
  mux/1 -> "pd{3,2}"/1
  "p{3}"/1 -> mux/1
